simulink model "ESTS_TFY_LafFAxle_test"  (R2023b)
settings: Solver=VariableStepAuto  StartTime=0.0  StopTime=10.0  RelTol=1e-3
libraries: ESTS_TFY_LatAxle x1
settings Model: Creator=blatak  LastModifiedBy=blatak

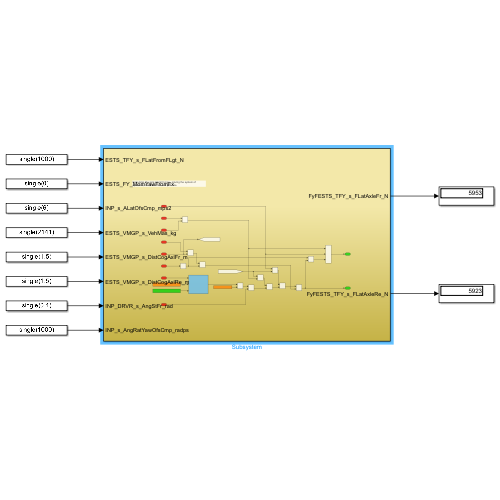
[thumbnail: Simulink's stored preview of the top-level diagram]
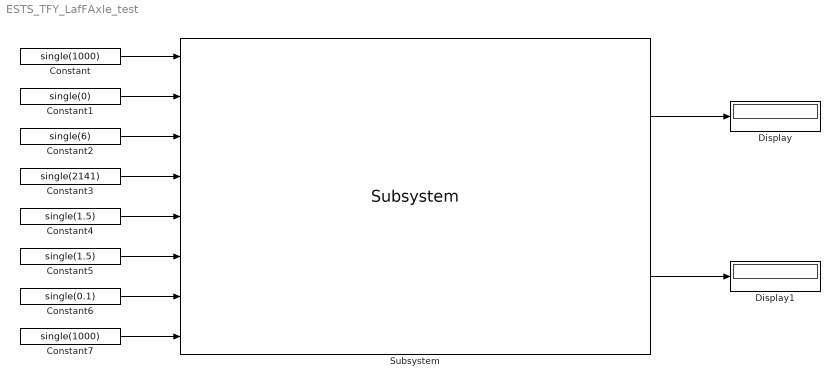
== system ESTS_TFY_LafFAxle_test ==
  Constant : Constant  Value=single(1000)
  Constant1 : Constant  Value=single(0)
  Constant2 : Constant  Value=single(6)
  Constant3 : Constant  Value=single(2141)
  Constant4 : Constant  Value=single(1.5)
  Constant5 : Constant  Value=single(1.5)
  Constant6 : Constant  Value=single(0.1)
  Constant7 : Constant  Value=single(1000)
  Display : Display
  Display1 : Display
  Subsystem : ESTS_TFY_LatAxle/Subsystem  SystemSampleTime=-1  VariantActivationTime=update diagram  AllowFlexibleInterface=on  Latency=0  AutoFrameSizeCalculation=off
  wires:
  Constant/1 -> Subsystem/1
  Constant1/1 -> Subsystem/2
  Constant2/1 -> Subsystem/3
  Constant3/1 -> Subsystem/4
  Constant4/1 -> Subsystem/5
  Constant5/1 -> Subsystem/6
  Constant6/1 -> Subsystem/7
  Constant7/1 -> Subsystem/8
  Subsystem/1 -> Display/1
  Subsystem/2 -> Display1/1
